simulink model "p3_car"  (R2025b)
settings: Solver=ode5  StartTime=0.0  StopTime=765  FixedStep=0.001  RelTol=1e-3
values from neighbouring files (symbols this model uses):
  DriveData = [ ... (first row only)    [initDriveCycle.m]
  Time = (0:1:765)'    [initDriveCycle.m]
undefined symbols (not defined in the file or in its folder): datBat, datCar
settings Model: Creator=dxego  LastModifiedBy=KI5UXW
settings OptimizationCC: ReuseModelBlockBuffer=off
settings DebuggingCC: AlgebraicLoopMsg=none
settings RTWCC: GPUComputeCapability=3.5

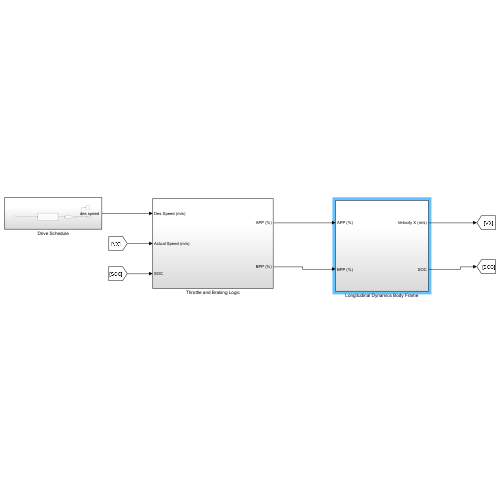
[thumbnail: Simulink's stored preview of the top-level diagram]
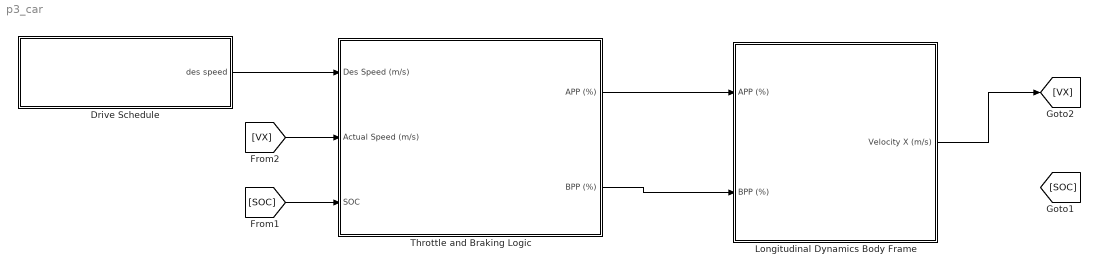
== system p3_car ==
  Drive Schedule : Subsystem
  Longitudinal Dynamics Body Frame : Subsystem
  "Throttle and Braking Logic " : Subsystem
  wires:
  "Throttle and Braking Logic "/1(APP (%)) -> Longitudinal Dynamics Body Frame/1(APP (%))
  "Throttle and Braking Logic "/2(BPP (%)) -> Longitudinal Dynamics Body Frame/2("BPP (%) ")
  Longitudinal Dynamics Body Frame/1(Velocity X (m/s)) -> [VX]
  Drive Schedule/1("des speed ") -> "Throttle and Braking Logic "/1("Des Speed (m/s) ")
  ? -> [SOC]
  [SOC] -> "Throttle and Braking Logic "/3(SOC)
  [VX] -> "Throttle and Braking Logic "/2(Actual Speed (m/s))

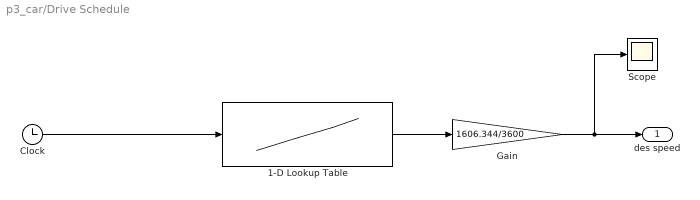
== system p3_car/Drive Schedule ==
  1-D Lookup Table : Lookup_n-D  NumberOfTableDimensions=1  BreakpointsForDimension1=Time  Table=DriveData  InternalRulePriority=Speed  RndMeth=Simplest
  Clock : Clock
  Gain : Gain  Gain=1606.344/3600
  Scope : Scope
      settings: ActiveDisplayYMinimum=-3.15  ActiveDisplayYMaximum=28.35  DataLoggingVariableName=ScopeData4
  "des speed " : Outport  VectorParamsAs1DForOutWhenUnconnected=off
  wires:
  Clock/1 -> 1-D Lookup Table/1
  1-D Lookup Table/1 -> Gain/1
  Gain/1 -> Scope/1, "des speed "/1

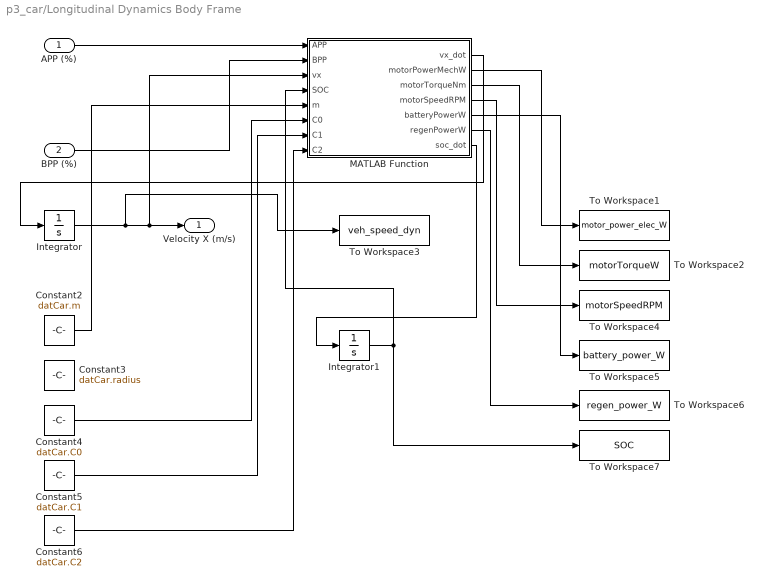
== system p3_car/Longitudinal Dynamics Body Frame ==
  APP (%) : Inport
  "BPP (%) " : Inport  Port=2
  Constant2 : Constant  Value=datCar.m
  Constant3 : Constant  Value=datCar.radius
  Constant4 : Constant  Value=datCar.C0
  Constant5 : Constant  Value=datCar.C1
  Constant6 : Constant  Value=datCar.C2
  Integrator : Integrator  InitialCondition=datCar.init.vx0
  Integrator1 : Integrator  InitialCondition=datBat.SOC_init
  MATLAB Function : MATLAB Function  TreatAsAtomicUnit=on
  To Workspace1 : ToWorkspace  VariableName=motor_power_elec_W  SaveFormat=Timeseries  SampleTime=-1
  To Workspace2 : ToWorkspace  VariableName=motorTorqueW  SaveFormat=Timeseries  SampleTime=-1
  To Workspace3 : ToWorkspace  VariableName=veh_speed_dyn  SaveFormat=Timeseries  SampleTime=-1
  To Workspace4 : ToWorkspace  VariableName=motorSpeedRPM  SaveFormat=Timeseries  SampleTime=-1
  To Workspace5 : ToWorkspace  VariableName=battery_power_W  SaveFormat=Timeseries  SampleTime=-1
  To Workspace6 : ToWorkspace  VariableName=regen_power_W  SaveFormat=Timeseries  SampleTime=-1
  To Workspace7 : ToWorkspace  VariableName=SOC  SaveFormat=Timeseries  SampleTime=-1
  Velocity X (m/s) : Outport
  wires:
  APP (%)/1 -> MATLAB Function/1(APP)
  "BPP (%) "/1 -> MATLAB Function/2(BPP)
  Integrator/1 -> To Workspace3/1, Velocity X (m/s)/1, MATLAB Function/3(vx)
  MATLAB Function/1(vx_dot) -> Integrator/1
  Constant2/1 -> MATLAB Function/5(m)
  Constant4/1 -> MATLAB Function/6(C0)
  Constant5/1 -> MATLAB Function/7(C1)
  Constant6/1 -> MATLAB Function/8(C2)
  MATLAB Function/2(motorPowerMechW) -> To Workspace1/1
  MATLAB Function/3(motorTorqueNm) -> To Workspace2/1
  MATLAB Function/4(motorSpeedRPM) -> To Workspace4/1
  MATLAB Function/7(soc_dot) -> Integrator1/1
  Integrator1/1 -> MATLAB Function/4(SOC), To Workspace7/1
  MATLAB Function/5(batteryPowerW) -> To Workspace5/1
  MATLAB Function/6(regenPowerW) -> To Workspace6/1

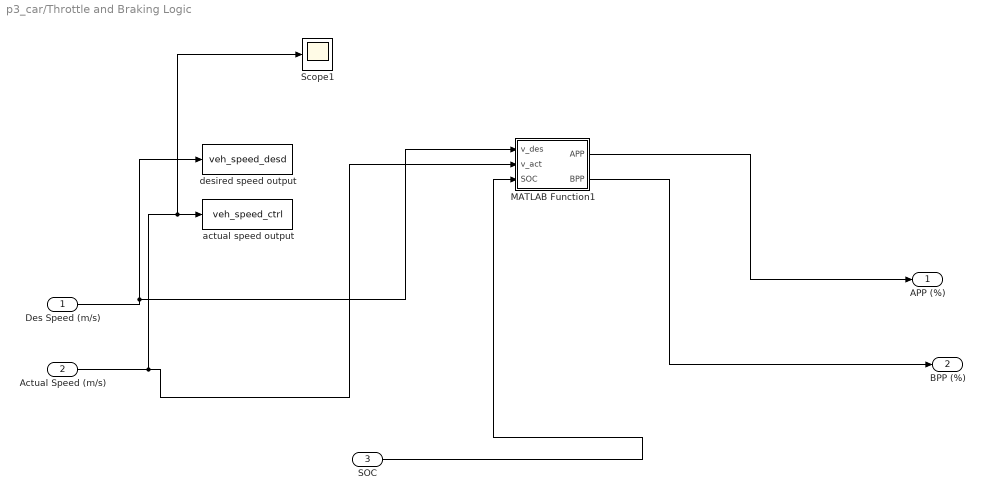
== system p3_car/Throttle and Braking Logic  ==
  "Des Speed (m/s) " : Inport
  Actual Speed (m/s) : Inport  Port=2
  SOC : Inport  Port=3
  MATLAB Function1 : MATLAB Function  TreatAsAtomicUnit=on
  Scope1 : Scope
      settings: ActiveDisplayYMinimum=-3.08288  ActiveDisplayYMaximum=27.75461
  actual speed output : ToWorkspace  VariableName=veh_speed_ctrl  SaveFormat=Timeseries  SampleTime=-1
  desired speed output : ToWorkspace  VariableName=veh_speed_desd  SaveFormat=Timeseries  SampleTime=-1
  APP (%) : Outport
  BPP (%) : Outport  Port=2
  wires:
  Actual Speed (m/s)/1 -> Scope1/1, actual speed output/1, MATLAB Function1/2(v_act)
  "Des Speed (m/s) "/1 -> MATLAB Function1/1(v_des), desired speed output/1
  SOC/1 -> MATLAB Function1/3(SOC)
  MATLAB Function1/1(APP) -> APP (%)/1
  MATLAB Function1/2(BPP) -> BPP (%)/1

== matlab function p3_car/Longitudinal Dynamics Body Frame/MATLAB Function ==
  data: APP input; vx_dot output; BPP input; vx input; SOC input; m input; C0 input; C1 input; C2 input; motorPowerMechW output; motorTorqueNm output; motorSpeedRPM output; batteryPowerW output; regenPowerW output; soc_dot output
function [vx_dot, motorPowerMechW, motorTorqueNm, motorSpeedRPM, batteryPowerW, regenPowerW, soc_dot] = ...
    fcn(APP, BPP, vx, SOC, m, C0, C1, C2)

% Constants
r_w = 0.3;                % wheel radius
gearRatio = 10.0;         % single speed ratio
FDRatio = 7.5;
FDeta = 0.95;

eta_drive = 0.92;
eta_regen = 0.70;

maxBrakeTorque = 50000;   % Nm
maxMotorTorque = 210;     % pick based on your scaled motor
maxRegenTorque = 120;     % capped regen torque

Q_C = 150 * 3600;         % battery charge in Coulombs
numSeries = 96;

% OCV lookup per cell
SOC_bp = [0 0.01 0.1 0.2 0.3 0.4 0.5 0.6 0.7 0.8 0.9 1.0];
OCV_bp = [0 3.1 3.55 3.68 3.74 3.76 3.78 3.85 3.9 3.95 4.08 4.15];

% Prevent divide-by-zero
vx_eff = max(vx, 0.001);

% ---------------- Motor speed ----------------
wheelSpeedRad = vx_eff / r_w;
motorSpeedRad = wheelSpeedRad * gearRatio * FDRatio;
motorSpeedRPM = motorSpeedRad * 60 / (2*pi);

% ---------------- Driver command ----------------
T_drive = (APP/100) * maxMotorTorque;

% Regen torque from brake command
T_regen = (BPP/100) * maxRegenTorque;

% Friction brake torque = total brake demand minus regen portion
T_brake_total = (BPP/100) * maxBrakeTorque;
T_brake_friction = max(T_brake_total - T_regen, 0);

% ---------------- Forces ----------------
F_drive = (T_drive * gearRatio * FDRatio * FDeta) / r_w;
F_regen = (T_regen * gearRatio * FDRatio * FDeta) / r_w;
F_brake = T_brake_friction / r_w;

F_drag = C0 + C1*vx_eff + C2*vx_eff^2;

% Net longitudinal force
Fx = F_drive - F_regen - F_brake - F_drag;

vx_dot = Fx / m;

% ---------------- Mechanical motor power ----------------
% positive when driving, negative when regen
motorTorqueNm = T_drive - T_regen;
motorPowerMechW = motorTorqueNm * motorSpeedRad;

% ---------------- Battery power ----------------
if motorPowerMechW >= 0
    batteryPowerW = motorPowerMechW / eta_drive;
    regenPowerW = 0;
else
    regenPowerW = -motorPowerMechW * eta_regen;
    batteryPowerW = -regenPowerW;  % negative means charging battery
end

% ---------------- SOC derivative ----------------
Vpack = interp1(SOC_bp, OCV_bp, min(max(SOC,0),1), 'linear', 'extrap') * numSeries;
Vpack = max(Vpack, 1);

Ibatt = batteryPowerW / Vpack;   % positive = discharging
soc_dot = -Ibatt / Q_C;

== matlab function p3_car/Throttle and Braking Logic /MATLAB Function1 ==
  data: v_des input; APP output; v_act input; SOC input; BPP output
function [APP,BPP] = fcn(v_des,v_act,SOC)
%#codegen

e = v_des - v_act;

Kp_throttle = 15;
Kp_brake = 20;

APP = 0;
BPP = 0;

if e >= 0
    APP = Kp_throttle * e;
    BPP = 0;
else
    APP = 0;
    BPP = Kp_brake * (-e);
end

APP = min(max(APP,0),100);
BPP = min(max(BPP,0),100);
